simulink model "data_acq_passiveV2"  (R2016b)
settings: Solver=FixedStepDiscrete  StartTime=0.0  StopTime=300  FixedStep=.001  RelTol=1e-3  EnableMultiTasking=on
values from neighbouring files (symbols this model uses):
  offset = [0 0]    [Calibration_Run_Script.m]    (also in DAQ_Run_Script.m; bias.m = signal)
undefined symbols (not defined in the file or in its folder): bit, fdesignblkfcn, gcbh, Standard
libraries: slrtlib x11, xpclib x6, canmsglib x5, simulink x5, xpcnilib x3
(part 1 of 2)
settings Model: SimulationMode=external  Creator=localadmin  LastModifiedBy=1108gotthem
settings SolverCC: EnableConcurrentExecution=on  AutoInsertRateTranBlk=on
settings DataIOCC: SaveFormat=Structure  SignalLoggingSaveFormat=ModelDataLogs
settings OptimizationCC: BlockReduction=off  OptimizeBlockIOStorage=off  BufferReuse=off  GlobalBufferReuse=off  ExpressionFolding=off  ExpressionDepthLimit=2147483647  LocalBlockOutputs=off
settings DebuggingCC: UnderspecifiedInitializationDetection=Classic  MergeDetectMultiDrivingBlocksExec=none  SolverPrmCheckMsg=warning  FcnCallInpInsideContextMsg=warning  StateNameClashWarn=warning  SFUnexpectedBacktrackingDiag=warning  SFNoUnconditionalDefaultTransitionDiag=warning  SFExecutionAtInitializationDiag=none
settings HardwareCC: ProdBitPerPointer=32  ProdBitPerSizeT=32  ProdBitPerPtrDiffT=32  ProdLargestAtomicFloat=None  ProdWordSize=32  ProdLongLongMode=on  ProdHWDeviceType=Generic->32-bit x86 compatible
settings ModelReferenceCC: PropagateSignalLabelsOutOfModel=off
settings RTWCC: SystemTargetFile=slrt.tlc  TemplateMakefile=slrt_default_tmf  Description=Simulink Real-Time  RTWCompilerOptimization=on
settings SimulinkRealTimeCC: RL32LogBufSizeModifier=10200000  xPCIRQSourceBoard=Speedgoat_IO331
settings ConfigComp: CovMetricSettings=dw  CovHtmlReporting=on  CovSaveCumulativeToWorkspaceVar=on  CovSaveSingleToWorkspaceVar=on  CovExternalEMLEnable=off

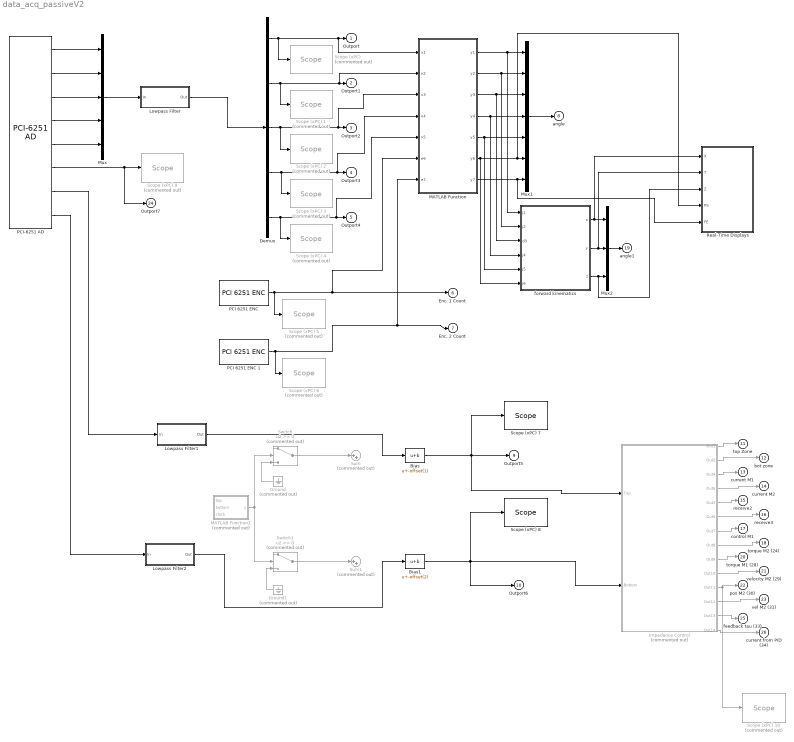
== system data_acq_passiveV2 ==
  Bias : Bias  Bias=-offset(1)
  Bias1 : Bias  Bias=-offset(2)
  Demux : Demux  Outputs=5
  Ground : Ground  Commented=on
  Ground1 : Ground  Commented=on
  Impedance Control : Subsystem  Commented=on
  Lowpass Filter : Subsystem  DialogController=fdesignblkfcn  InitFcn=fdesignblkfcn(gcbh, {'InitFcn'});  mask(Lowpass Filter){}
      mask help: Design a lowpass filter
      settings: CopyFcn=fdesignblkfcn(gcbh, {'CopyFcn'});
      mask Help: helpview(mapfilelocation('dsp'), 'dsplowpassfilter');
      mask Display: disp('Lowpass')
  Lowpass Filter1 : Subsystem  DialogController=fdesignblkfcn  InitFcn=fdesignblkfcn(gcbh, {'InitFcn'});  mask(Lowpass Filter){}
      mask help: Design a lowpass filter
      settings: CopyFcn=fdesignblkfcn(gcbh, {'CopyFcn'});
      mask Help: helpview(mapfilelocation('dsp'), 'dsplowpassfilter');
      mask Display: disp('Lowpass')
  Lowpass Filter2 : Subsystem  DialogController=fdesignblkfcn  InitFcn=fdesignblkfcn(gcbh, {'InitFcn'});  mask(Lowpass Filter){}
      mask help: Design a lowpass filter
      settings: CopyFcn=fdesignblkfcn(gcbh, {'CopyFcn'});
      mask Help: helpview(mapfilelocation('dsp'), 'dsplowpassfilter');
      mask Display: disp('Lowpass')
  MATLAB Function : MATLAB Function  TreatAsAtomicUnit=on
  MATLAB Function1 : MATLAB Function  Commented=on  TreatAsAtomicUnit=on
  Mux : Mux  Inputs=5
  Mux1 : Mux  Inputs=7
  Mux2 : Mux  Inputs=3
  "PCI 6251 ENC " : xpcnilib/Incremental Encoder/PCI 6251 ENC   channel=1  countMode=Quadrature Mode x4  initCount=0  reload=off  indexPhase=A low B low  filter=None  sampleTime=0.001  slot=-1
  PCI 6251 ENC 1 : xpcnilib/Incremental Encoder/PCI 6251 ENC   channel=0  countMode=Quadrature Mode x4  initCount=0  reload=off  indexPhase=A low B low  filter=None  sampleTime=0.001  slot=-1
  PCI-6251 AD : xpcnilib/A//D/M Series/PCI-6251 AD  channel=[1,2,3,4,5,6,7,8]  range=[10,10,10,10,10,10,10,10]  coupling=[1,1,1,1,1,1,2,2]  scantime=5e-6  sampletime=0.001  slot=-1
  "Real-Time Displays " : Subsystem
  "Scope (xPC) " : slrtlib/Displays and Logging/Scope   Commented=on  scopeno=6  scopetype=Target  autostart=on  viewmode=Graphical rolling  formatstr='%15.6f'  grid=on  ylimits=[7,10]  nosamples=15001  noprepostsamples=0  interleave=1  triggermode=FreeRun  triggersignal=1  trigsignalfromport=off  triggerlevel=0.0  triggerslope=Either  triggerscope=1  triggersample=0  filename=data.dat  mode=Lazy  writesize=512  autorestart=off  dynamicfilemode=off  maxwritefilesize=512*1024^2
  Scope (xPC) 1 : slrtlib/Displays and Logging/Scope   Commented=on  scopeno=1  scopetype=Target  autostart=on  viewmode=Graphical rolling  formatstr='%15.6f'  grid=on  ylimits=[5,9]  nosamples=15001  noprepostsamples=0  interleave=1  triggermode=FreeRun  triggersignal=1  trigsignalfromport=off  triggerlevel=0.0  triggerslope=Either  triggerscope=1  triggersample=0  filename=data.dat  mode=Lazy  writesize=512  autorestart=off  dynamicfilemode=off  maxwritefilesize=512*1024^2
  Scope (xPC) 10 : slrtlib/Displays and Logging/Scope   Commented=on  scopeno=5  scopetype=Target  autostart=on  viewmode=Graphical rolling  formatstr='%15.6f'  grid=on  ylimits=[-250,250]  nosamples=15001  noprepostsamples=0  interleave=1  triggermode=FreeRun  triggersignal=1  trigsignalfromport=off  triggerlevel=0.0  triggerslope=Either  triggerscope=1  triggersample=0  filename=data.dat  mode=Lazy  writesize=512  autorestart=off  dynamicfilemode=off  maxwritefilesize=512*1024^2
  Scope (xPC) 2 : slrtlib/Displays and Logging/Scope   Commented=on  scopeno=2  scopetype=Target  autostart=on  viewmode=Graphical rolling  formatstr='%15.6f'  grid=on  ylimits=[0,10]  nosamples=15001  noprepostsamples=0  interleave=1  triggermode=FreeRun  triggersignal=1  trigsignalfromport=off  triggerlevel=0.0  triggerslope=Either  triggerscope=1  triggersample=0  filename=data.dat  mode=Lazy  writesize=512  autorestart=off  dynamicfilemode=off  maxwritefilesize=512*1024^2
  Scope (xPC) 3 : slrtlib/Displays and Logging/Scope   Commented=on  scopeno=3  scopetype=Target  autostart=on  viewmode=Graphical rolling  formatstr='%15.6f'  grid=on  ylimits=[4.5,8.5]  nosamples=15001  noprepostsamples=0  interleave=1  triggermode=FreeRun  triggersignal=1  trigsignalfromport=off  triggerlevel=0.0  triggerslope=Either  triggerscope=1  triggersample=0  filename=data.dat  mode=Lazy  writesize=512  autorestart=off  dynamicfilemode=off  maxwritefilesize=512*1024^2
  Scope (xPC) 4 : slrtlib/Displays and Logging/Scope   Commented=on  scopeno=7  scopetype=Target  autostart=on  viewmode=Graphical rolling  formatstr='%15.6f'  grid=on  ylimits=[5,9]  nosamples=15001  noprepostsamples=0  interleave=1  triggermode=FreeRun  triggersignal=1  trigsignalfromport=off  triggerlevel=0.0  triggerslope=Either  triggerscope=1  triggersample=0  filename=data.dat  mode=Lazy  writesize=512  autorestart=off  dynamicfilemode=off  maxwritefilesize=512*1024^2
  Scope (xPC) 5 : slrtlib/Displays and Logging/Scope   Commented=on  scopeno=4  scopetype=Target  autostart=on  viewmode=Graphical rolling  formatstr='%15.6f'  grid=on  ylimits=[-15000,15000]  nosamples=15001  noprepostsamples=0  interleave=1  triggermode=FreeRun  triggersignal=1  trigsignalfromport=off  triggerlevel=0.0  triggerslope=Either  triggerscope=1  triggersample=0  filename=data.dat  mode=Lazy  writesize=512  autorestart=off  dynamicfilemode=off  maxwritefilesize=512*1024^2
  Scope (xPC) 6 : slrtlib/Displays and Logging/Scope   Commented=on  scopeno=5  scopetype=Target  autostart=on  viewmode=Graphical rolling  formatstr='%15.6f'  grid=on  ylimits=[-40000,40000]  nosamples=15001  noprepostsamples=0  interleave=1  triggermode=FreeRun  triggersignal=1  trigsignalfromport=off  triggerlevel=0.0  triggerslope=Either  triggerscope=1  triggersample=0  filename=data.dat  mode=Lazy  writesize=512  autorestart=off  dynamicfilemode=off  maxwritefilesize=512*1024^2
  Scope (xPC) 7 : slrtlib/Displays and Logging/Scope   scopeno=8  scopetype=Target  autostart=on  viewmode=Graphical rolling  formatstr='%15.6f'  grid=on  ylimits=[-1,1]  nosamples=20001  noprepostsamples=0  interleave=1  triggermode=FreeRun  triggersignal=1  trigsignalfromport=off  triggerlevel=0.0  triggerslope=Either  triggerscope=1  triggersample=0  filename=data.dat  mode=Lazy  writesize=512  autorestart=off  dynamicfilemode=off  maxwritefilesize=512*1024^2
  Scope (xPC) 8 : slrtlib/Displays and Logging/Scope   scopeno=9  scopetype=Target  autostart=on  viewmode=Graphical rolling  formatstr='%15.6f'  grid=on  ylimits=[-1,1]  nosamples=20001  noprepostsamples=0  interleave=1  triggermode=FreeRun  triggersignal=1  trigsignalfromport=off  triggerlevel=0.0  triggerslope=Either  triggerscope=1  triggersample=0  filename=data.dat  mode=Lazy  writesize=512  autorestart=off  dynamicfilemode=off  maxwritefilesize=512*1024^2
  Scope (xPC) 9 : slrtlib/Displays and Logging/Scope   Commented=on  scopeno=2  scopetype=Target  autostart=on  viewmode=Graphical rolling  formatstr='%15.6f'  grid=on  ylimits=[0,10]  nosamples=15001  noprepostsamples=0  interleave=1  triggermode=FreeRun  triggersignal=1  trigsignalfromport=off  triggerlevel=0.0  triggerslope=Either  triggerscope=1  triggersample=0  filename=data.dat  mode=Lazy  writesize=512  autorestart=off  dynamicfilemode=off  maxwritefilesize=512*1024^2
  Sum : Sum  Commented=on  Inputs=|++
  Sum1 : Sum  Commented=on  Inputs=|++
  Switch : Switch  Commented=on
  Switch1 : Switch  Commented=on
  forward kinematics : MATLAB Function  TreatAsAtomicUnit=on
  Outport : Outport  InitialOutput=0
  Outport1 : Outport  Port=2  InitialOutput=0
  Outport2 : Outport  Port=3  InitialOutput=0
  Outport3 : Outport  Port=4  InitialOutput=0
  Outport4 : Outport  Port=5  InitialOutput=0
  Enc. 1 Count : Outport  Port=6  InitialOutput=0
  Enc. 2 Count : Outport  Port=7  InitialOutput=0
  angle : Outport  Port=8  InitialOutput=0
  Outport5 : Outport  Port=9  InitialOutput=0
  Outport6 : Outport  Port=10  InitialOutput=0
  top Zone : Outport  Port=11  InitialOutput=0
  bot zone : Outport  Port=12  InitialOutput=0
  current M1 : Outport  Port=13  InitialOutput=0
  current M2 : Outport  Port=14  InitialOutput=0
  receive2 : Outport  Port=15  InitialOutput=0
  receive3 : Outport  Port=16  InitialOutput=0
  control M1 : Outport  Port=17  InitialOutput=0
  torque M2 (24) : Outport  Port=18  InitialOutput=0
  angle1 : Outport  Port=19  InitialOutput=0
  torque M1 (28) : Outport  Port=20  InitialOutput=0
  velocity M2 (29) : Outport  Port=21  InitialOutput=0
  pos M2 (30) : Outport  Port=22  InitialOutput=0
  vel M2 (31) : Outport  Port=23  InitialOutput=0
  Outport7 : Outport  Port=24  InitialOutput=0
  feedback tau (33) : Outport  Port=25  InitialOutput=0
  current from PID (34) : Outport  Port=26  InitialOutput=0
  wires:
  PCI-6251 AD/1 -> Mux/1
  PCI-6251 AD/2 -> Mux/2
  PCI-6251 AD/3 -> Mux/3
  PCI-6251 AD/4 -> Mux/4
  Demux/1 -> "Scope (xPC) "/1, MATLAB Function/1(v1), Outport/1
  Lowpass Filter/1(Out) -> Demux/1
  MATLAB Function/1(y1) -> forward kinematics/1(j1), Mux1/1
  MATLAB Function/2(y2) -> forward kinematics/2(j2), Mux1/2
  MATLAB Function/3(y3) -> forward kinematics/3(d3), Mux1/3
  MATLAB Function/4(y4) -> forward kinematics/4(j4), Mux1/4
  MATLAB Function/5(y5) -> forward kinematics/5(j5), Mux1/5
  Mux1/1 -> angle/1
  MATLAB Function/6(y6) -> forward kinematics/6(j6), "Real-Time Displays "/4(PS), Mux1/6
  MATLAB Function/7(y7) -> "Real-Time Displays "/5(FE), Mux1/7
  PCI-6251 AD/5 -> Mux/5
  Mux/1 -> Lowpass Filter/1(In)
  Demux/2 -> Scope (xPC) 1/1, MATLAB Function/2(v2), Outport1/1
  Demux/3 -> Scope (xPC) 2/1, MATLAB Function/3(v3), Outport2/1
  Demux/4 -> Scope (xPC) 3/1, MATLAB Function/4(v4), Outport3/1
  Demux/5 -> Scope (xPC) 4/1, Outport4/1, MATLAB Function/5(v5)
  PCI 6251 ENC 1/1 -> MATLAB Function/7(e7), Enc. 2 Count/1, Scope (xPC) 6/1
  "PCI 6251 ENC "/1 -> Scope (xPC) 5/1, MATLAB Function/6(e6), Enc. 1 Count/1
  Impedance Control/1(Out1) -> top Zone/1
  Impedance Control/2(Out2) -> bot zone/1
  Impedance Control/3(Out4) -> current M1/1
  Impedance Control/4(Out6) -> current M2/1
  Impedance Control/5(Out3) -> receive2/1
  Impedance Control/6(Out5) -> receive3/1
  Impedance Control/7(Out7) -> control M1/1
  Impedance Control/8(Out8) -> torque M2 (24)/1
  forward kinematics/1(x) -> "Real-Time Displays "/1(X), Mux2/1
  forward kinematics/2(y) -> "Real-Time Displays "/2(Y), Mux2/2
  forward kinematics/3(z) -> "Real-Time Displays "/3(Z), Mux2/3
  Mux2/1 -> angle1/1
  Impedance Control/9(Out9) -> torque M1 (28)/1
  Impedance Control/10(Out10) -> velocity M2 (29)/1
  Impedance Control/12(Out12) -> vel M2 (31)/1
  MATLAB Function1/1(y) -> Switch/2, Switch1/2
  Ground/1 -> Switch/3
  Switch/1 -> Sum/1
  Ground1/1 -> Switch1/3
  Switch1/1 -> Sum1/1
  Bias/1 -> Impedance Control/1(Top), Scope (xPC) 7/1, Outport5/1
  Bias1/1 -> Scope (xPC) 8/1, Outport6/1, Impedance Control/2(Bottom)
  PCI-6251 AD/6 -> Outport7/1, Scope (xPC) 9/1
  Impedance Control/11(Out11) -> Scope (xPC) 10/1, pos M2 (30)/1
  Impedance Control/13(Out13) -> feedback tau (33)/1
  Impedance Control/14(Out14) -> current from PID (34)/1
  PCI-6251 AD/7 -> Lowpass Filter1/1(In)
  Lowpass Filter1/1(Out) -> Bias/1
  PCI-6251 AD/8 -> Lowpass Filter2/1(In)
  Lowpass Filter2/1(Out) -> Bias1/1

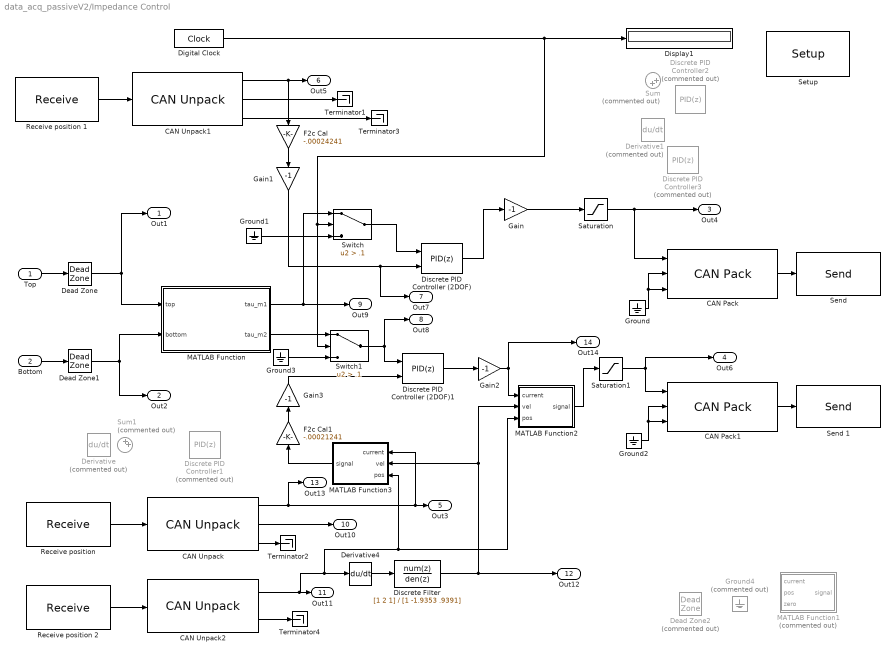
== system data_acq_passiveV2/Impedance Control ==
  Top : Inport
  Bottom : Inport  Port=2
  CAN Pack : canmsglib/CAN Pack  MsgList=(none)  MsgName=CAN Msg  MsgIDType=Standard (11-bit identifier)  MsgIdentifier=hex2dec('202')  MsgLength=8  SignalInfo=current$0$16$1$1$1$0$1$0$-Inf$Inf$#null$16$16$1$1$1$0$1$0$-Inf$Inf$#null2$32$32$1$1$1$0$1$0$-Inf$Inf$#  NSignals=3  StartBits=str2num('[int32(0);int32(16);int32(32)]')  SignalSizes=str2num('[int32(16);int32(16);int32(32)]')  ByteOrders=str2num('[int32(1);int32(1);int32(1)]')  DataTypes=str2num('[int32(1);int32(1);int32(1)]')  MultiplexTypes=str2num('[int32(1);int32(1);int32(1)]')  MultiplexValues=str2num('[double(0);double(0);double(0)]')  Factors=str2num('[double(1);double(1);double(1)]')  Offsets=str2num('[double(0);double(0);double(0)]')  Minimums=str2num('[double(-Inf);double(-Inf);double(-Inf)]')  Maximums=str2num('[double(Inf);double(Inf);double(Inf)]')  Remote=off
      settings: DataFormat=manually specified signals
  CAN Pack1 : canmsglib/CAN Pack  MsgList=(none)  MsgName=CAN Msg  MsgIDType=Standard (11-bit identifier)  MsgIdentifier=hex2dec('201')  MsgLength=8  SignalInfo=current$0$16$1$1$1$0$1$0$-Inf$Inf$#null$16$16$1$1$1$0$1$0$-Inf$Inf$#null2$32$32$1$1$1$0$1$0$-Inf$Inf$#  NSignals=3  StartBits=str2num('[int32(0);int32(16);int32(32)]')  SignalSizes=str2num('[int32(16);int32(16);int32(32)]')  ByteOrders=str2num('[int32(1);int32(1);int32(1)]')  DataTypes=str2num('[int32(1);int32(1);int32(1)]')  MultiplexTypes=str2num('[int32(1);int32(1);int32(1)]')  MultiplexValues=str2num('[double(0);double(0);double(0)]')  Factors=str2num('[double(1);double(1);double(1)]')  Offsets=str2num('[double(0);double(0);double(0)]')  Minimums=str2num('[double(-Inf);double(-Inf);double(-Inf)]')  Maximums=str2num('[double(Inf);double(Inf);double(Inf)]')  Remote=off
      settings: DataFormat=manually specified signals
  CAN Unpack : canmsglib/CAN Unpack  MsgList=(none)  MsgName=CAN Msg  MsgIDType=Standard (11-bit identifier)  MsgIdentifier=hex2dec('181')  MsgLength=8  SignalInfo=Current$0$16$1$1$1$0$1$0$-Inf$Inf$#vel$16$32$1$2$1$0$1$0$-Inf$Inf$#null2$48$16$1$1$1$0$1$0$-Inf$Inf$#  NSignals=3  IDPort=off  TimestampPort=off  ErrorPort=off  RemotePort=off  LengthPort=off  StatusPort=off  StartBits=str2num('[int32(0);int32(16);int32(48)]')  SignalSizes=str2num('[int32(16);int32(32);int32(16)]')  ByteOrders=str2num('[int32(1);int32(1);int32(1)]')  DataTypes=str2num('[int32(1);int32(2);int32(1)]')  MultiplexTypes=str2num('[int32(1);int32(1);int32(1)]')  MultiplexValues=str2num('[double(0);double(0);double(0)]')  Factors=str2num('[double(1);double(1);double(1)]')  Offsets=str2num('[double(0);double(0);double(0)]')  Minimums=str2num('[double(-Inf);double(-Inf);double(-Inf)]')  Maximums=str2num('[double(Inf);double(Inf);double(Inf)]')
  CAN Unpack1 : canmsglib/CAN Unpack  MsgList=(none)  MsgName=CAN Msg  MsgIDType=Standard (11-bit identifier)  MsgIdentifier=hex2dec('182')  MsgLength=8  SignalInfo=Current$0$16$1$1$1$0$1$0$-Inf$Inf$#null$16$32$1$2$1$0$1$0$-Inf$Inf$#null2$48$16$1$1$1$0$1$0$-Inf$Inf$#  NSignals=3  IDPort=off  TimestampPort=off  ErrorPort=off  RemotePort=off  LengthPort=off  StatusPort=off  StartBits=str2num('[int32(0);int32(16);int32(48)]')  SignalSizes=str2num('[int32(16);int32(32);int32(16)]')  ByteOrders=str2num('[int32(1);int32(1);int32(1)]')  DataTypes=str2num('[int32(1);int32(2);int32(1)]')  MultiplexTypes=str2num('[int32(1);int32(1);int32(1)]')  MultiplexValues=str2num('[double(0);double(0);double(0)]')  Factors=str2num('[double(1);double(1);double(1)]')  Offsets=str2num('[double(0);double(0);double(0)]')  Minimums=str2num('[double(-Inf);double(-Inf);double(-Inf)]')  Maximums=str2num('[double(Inf);double(Inf);double(Inf)]')
  CAN Unpack2 : canmsglib/CAN Unpack  MsgList=(none)  MsgName=CAN Msg  MsgIDType=Standard (11-bit identifier)  MsgIdentifier=hex2dec('281')  MsgLength=8  SignalInfo=pos$0$32$1$1$1$0$1$0$-Inf$Inf$#null$32$32$1$2$1$0$1$0$-Inf$Inf$#  NSignals=2  IDPort=off  TimestampPort=off  ErrorPort=off  RemotePort=off  LengthPort=off  StatusPort=off  StartBits=str2num('[int32(0);int32(32)]')  SignalSizes=str2num('[int32(32);int32(32)]')  ByteOrders=str2num('[int32(1);int32(1)]')  DataTypes=str2num('[int32(1);int32(2)]')  MultiplexTypes=str2num('[int32(1);int32(1)]')  MultiplexValues=str2num('[double(0);double(0)]')  Factors=str2num('[double(1);double(1)]')  Offsets=str2num('[double(0);double(0)]')  Minimums=str2num('[double(-Inf);double(-Inf)]')  Maximums=str2num('[double(Inf);double(Inf)]')
  Dead Zone : DeadZone  LowerValue=-.05  UpperValue=.05  SampleTime=.001  SaturateOnIntegerOverflow=on
  Dead Zone1 : DeadZone  LowerValue=-.05  UpperValue=.05  SampleTime=.001  SaturateOnIntegerOverflow=on
  Dead Zone2 : DeadZone  Commented=on  LowerValue=-4e4  UpperValue=4e4  SampleTime=.001  SaturateOnIntegerOverflow=on
  Derivative : Derivative  Commented=on
  Derivative1 : Derivative  Commented=on
  Derivative4 : Derivative
  Digital Clock : DigitalClock  SampleTime=.001
  Discrete Filter : DiscreteFilter  Numerator=[1 2 1]  Denominator=[1 -1.9353 .9391]  SampleTime=.001
  Discrete PID Controller (2DOF) : simulink/Continuous/PID Controller (2DOF)  Controller=PID  TimeDomain=Discrete-time  SampleTime=.001  IntegratorMethod=Forward Euler  FilterMethod=Forward Euler  Form=Parallel  P=-206.434175056882  I=-412868.350113764  D=0  N=100  b=1  c=1  InitialConditionSource=internal  InitialConditionForIntegrator=0  InitialConditionForFilter=0  ExternalReset=none  LimitOutput=off  UpperSaturationLimit=inf  LowerSaturationLimit=-inf  LinearizeAsGain=off  AntiWindupMode=none  Kb=1  TrackingMode=off  Kt=1  PParamMin=[]  PParamMax=[]  IParamMin=[]  IParamMax=[]  DParamMin=[]  DParamMax=[]  NParamMin=[]  NParamMax=[]  bParamMin=[]  bParamMax=[]  cParamMin=[]  cParamMax=[]  KbParamMin=[]  KbParamMax=[]  KtParamMin=[]  KtParamMax=[]  POutMin=[]  POutMax=[]  IOutMin=[]  IOutMax=[]  DOutMin=[]  DOutMax=[]  NOutMin=[]  NOutMax=[]  bOutMin=[]  bOutMax=[]  cOutMin=[]  cOutMax=[]  KbOutMin=[]  KbOutMax=[]  KtOutMin=[]  KtOutMax=[]  IntegratorOutMin=[]  IntegratorOutMax=[]  FilterOutMin=[]  FilterOutMax=[]  SumOutMin=[]  SumOutMax=[]  Sum1OutMin=[]  Sum1OutMax=[]  Sum2OutMin=[]  Sum2OutMax=[]  Sum3OutMin=[]  Sum3OutMax=[]  SumI1OutMin=[]  SumI1OutMax=[]  SumI2OutMin=[]  SumI2OutMax=[]  SumI3OutMin=[]  SumI3OutMax=[]  SumDOutMin=[]  SumDOutMax=[]  SaturationOutMin=[]  SaturationOutMax=[]  IntegratorContinuousStateAttributes=''  IntegratorStateMustResolveToSignalObject=off  IntegratorRTWStateStorageClass=Auto  FilterContinuousStateAttributes=''  FilterStateMustResolveToSignalObject=off  FilterRTWStateStorageClass=Auto
  Discrete PID Controller (2DOF)1 : simulink/Continuous/PID Controller (2DOF)  Controller=PID  TimeDomain=Discrete-time  SampleTime=.001  IntegratorMethod=Forward Euler  FilterMethod=Forward Euler  Form=Parallel  P=-235.590171722324  I=-471180.343444648  D=0  N=100  b=1  c=1  InitialConditionSource=internal  InitialConditionForIntegrator=0  InitialConditionForFilter=0  ExternalReset=none  LimitOutput=off  UpperSaturationLimit=inf  LowerSaturationLimit=-inf  LinearizeAsGain=off  AntiWindupMode=none  Kb=1  TrackingMode=off  Kt=1  PParamMin=[]  PParamMax=[]  IParamMin=[]  IParamMax=[]  DParamMin=[]  DParamMax=[]  NParamMin=[]  NParamMax=[]  bParamMin=[]  bParamMax=[]  cParamMin=[]  cParamMax=[]  KbParamMin=[]  KbParamMax=[]  KtParamMin=[]  KtParamMax=[]  POutMin=[]  POutMax=[]  IOutMin=[]  IOutMax=[]  DOutMin=[]  DOutMax=[]  NOutMin=[]  NOutMax=[]  bOutMin=[]  bOutMax=[]  cOutMin=[]  cOutMax=[]  KbOutMin=[]  KbOutMax=[]  KtOutMin=[]  KtOutMax=[]  IntegratorOutMin=[]  IntegratorOutMax=[]  FilterOutMin=[]  FilterOutMax=[]  SumOutMin=[]  SumOutMax=[]  Sum1OutMin=[]  Sum1OutMax=[]  Sum2OutMin=[]  Sum2OutMax=[]  Sum3OutMin=[]  Sum3OutMax=[]  SumI1OutMin=[]  SumI1OutMax=[]  SumI2OutMin=[]  SumI2OutMax=[]  SumI3OutMin=[]  SumI3OutMax=[]  SumDOutMin=[]  SumDOutMax=[]  SaturationOutMin=[]  SaturationOutMax=[]  IntegratorContinuousStateAttributes=''  IntegratorStateMustResolveToSignalObject=off  IntegratorRTWStateStorageClass=Auto  FilterContinuousStateAttributes=''  FilterStateMustResolveToSignalObject=off  FilterRTWStateStorageClass=Auto
  Discrete PID Controller1 : simulink/Continuous/PID Controller  Commented=on  Controller=PID  TimeDomain=Discrete-time  SampleTime=.001  IntegratorMethod=Forward Euler  FilterMethod=Forward Euler  Form=Parallel  P=-1.8  I=-4000  D=0  N=100  InitialConditionSource=internal  InitialConditionForIntegrator=0  InitialConditionForFilter=0  ExternalReset=none  LimitOutput=off  UpperSaturationLimit=inf  LowerSaturationLimit=-inf  LinearizeAsGain=off  AntiWindupMode=none  Kb=1  TrackingMode=off  Kt=1  PParamMin=[]  PParamMax=[]  IParamMin=[]  IParamMax=[]  DParamMin=[]  DParamMax=[]  NParamMin=[]  NParamMax=[]  KbParamMin=[]  KbParamMax=[]  KtParamMin=[]  KtParamMax=[]  POutMin=[]  POutMax=[]  IOutMin=[]  IOutMax=[]  DOutMin=[]  DOutMax=[]  NOutMin=[]  NOutMax=[]  KbOutMin=[]  KbOutMax=[]  KtOutMin=[]  KtOutMax=[]  IntegratorOutMin=[]  IntegratorOutMax=[]  FilterOutMin=[]  FilterOutMax=[]  SumOutMin=[]  SumOutMax=[]  SumI1OutMin=[]  SumI1OutMax=[]  SumI2OutMin=[]  SumI2OutMax=[]  SumI3OutMin=[]  SumI3OutMax=[]  SumDOutMin=[]  SumDOutMax=[]  SaturationOutMin=[]  SaturationOutMax=[]  IntegratorContinuousStateAttributes=''  IntegratorStateMustResolveToSignalObject=off  IntegratorRTWStateStorageClass=Auto  FilterContinuousStateAttributes=''  FilterStateMustResolveToSignalObject=off  FilterRTWStateStorageClass=Auto
  Discrete PID Controller2 : simulink/Continuous/PID Controller  Commented=on  Controller=PID  TimeDomain=Discrete-time  SampleTime=.001  IntegratorMethod=Forward Euler  FilterMethod=Forward Euler  Form=Parallel  P=10  I=500  D=2  N=1  InitialConditionSource=internal  InitialConditionForIntegrator=0  InitialConditionForFilter=0  ExternalReset=none  LimitOutput=off  UpperSaturationLimit=inf  LowerSaturationLimit=-inf  LinearizeAsGain=off  AntiWindupMode=none  Kb=1  TrackingMode=off  Kt=1  PParamMin=[]  PParamMax=[]  IParamMin=[]  IParamMax=[]  DParamMin=[]  DParamMax=[]  NParamMin=[]  NParamMax=[]  KbParamMin=[]  KbParamMax=[]  KtParamMin=[]  KtParamMax=[]  POutMin=[]  POutMax=[]  IOutMin=[]  IOutMax=[]  DOutMin=[]  DOutMax=[]  NOutMin=[]  NOutMax=[]  KbOutMin=[]  KbOutMax=[]  KtOutMin=[]  KtOutMax=[]  IntegratorOutMin=[]  IntegratorOutMax=[]  FilterOutMin=[]  FilterOutMax=[]  SumOutMin=[]  SumOutMax=[]  SumI1OutMin=[]  SumI1OutMax=[]  SumI2OutMin=[]  SumI2OutMax=[]  SumI3OutMin=[]  SumI3OutMax=[]  SumDOutMin=[]  SumDOutMax=[]  SaturationOutMin=[]  SaturationOutMax=[]  IntegratorContinuousStateAttributes=''  IntegratorStateMustResolveToSignalObject=off  IntegratorRTWStateStorageClass=Auto  FilterContinuousStateAttributes=''  FilterStateMustResolveToSignalObject=off  FilterRTWStateStorageClass=Auto
  Discrete PID Controller3 : simulink/Continuous/PID Controller  Commented=on  Controller=PID  TimeDomain=Discrete-time  SampleTime=.001  IntegratorMethod=Forward Euler  FilterMethod=Forward Euler  Form=Parallel  P=-1.8  I=-4000  D=0  N=100  InitialConditionSource=internal  InitialConditionForIntegrator=0  InitialConditionForFilter=0  ExternalReset=none  LimitOutput=off  UpperSaturationLimit=inf  LowerSaturationLimit=-inf  LinearizeAsGain=off  AntiWindupMode=none  Kb=1  TrackingMode=off  Kt=1  PParamMin=[]  PParamMax=[]  IParamMin=[]  IParamMax=[]  DParamMin=[]  DParamMax=[]  NParamMin=[]  NParamMax=[]  KbParamMin=[]  KbParamMax=[]  KtParamMin=[]  KtParamMax=[]  POutMin=[]  POutMax=[]  IOutMin=[]  IOutMax=[]  DOutMin=[]  DOutMax=[]  NOutMin=[]  NOutMax=[]  KbOutMin=[]  KbOutMax=[]  KtOutMin=[]  KtOutMax=[]  IntegratorOutMin=[]  IntegratorOutMax=[]  FilterOutMin=[]  FilterOutMax=[]  SumOutMin=[]  SumOutMax=[]  SumI1OutMin=[]  SumI1OutMax=[]  SumI2OutMin=[]  SumI2OutMax=[]  SumI3OutMin=[]  SumI3OutMax=[]  SumDOutMin=[]  SumDOutMax=[]  SaturationOutMin=[]  SaturationOutMax=[]  IntegratorContinuousStateAttributes=''  IntegratorStateMustResolveToSignalObject=off  IntegratorRTWStateStorageClass=Auto  FilterContinuousStateAttributes=''  FilterStateMustResolveToSignalObject=off  FilterRTWStateStorageClass=Auto
  Display1 : Display
      settings: Format=hex (Stored Integer)
  F2c Cal : Gain  Gain=-.00024241  SampleTime=.001
  F2c Cal1 : Gain  Gain=-.00021241  SampleTime=.001
  Gain{,1..3} (4 alike) : Gain  Gain=-1
  Ground{,1..3} (4 alike) : Ground
  Ground4 : Ground  Commented=on
  MATLAB Function : MATLAB Function  TreatAsAtomicUnit=on
  MATLAB Function1 : MATLAB Function  Commented=on  TreatAsAtomicUnit=on
  MATLAB Function2 : MATLAB Function  TreatAsAtomicUnit=on
  MATLAB Function3 : MATLAB Function  TreatAsAtomicUnit=on
  "Receive position " : xpclib/CAN/Softing/CAN-AC2-PCI SJA 1000/Receive   board=1  canPort=CAN 1  range=Standard (11-bit)  ids=hex2dec('181')  lengths=8  output=CAN_MESSAGE data type  inten=off  ts=0.001  ididx=[0]
  Receive position 1 : xpclib/CAN/Softing/CAN-AC2-PCI SJA 1000/Receive   board=1  canPort=CAN 1  range=Standard (11-bit)  ids=hex2dec('182')  lengths=8  output=CAN_MESSAGE data type  inten=off  ts=0.001  ididx=[1]
  Receive position 2 : xpclib/CAN/Softing/CAN-AC2-PCI SJA 1000/Receive   board=1  canPort=CAN 1  range=Standard (11-bit)  ids=hex2dec('281')  lengths=8  output=CAN_MESSAGE data type  inten=off  ts=0.001  ididx=[2]
  Saturation : Saturate  UpperLimit=1700  LowerLimit=-1700  LinearizeAsGain=off  SampleTime=.001
  Saturation1 : Saturate  UpperLimit=1700  LowerLimit=-1700  LinearizeAsGain=off
  "Send " : xpclib/CAN/Softing/CAN-AC2-PCI SJA 1000/Send   board=1  canPort=CAN 1  range=Standard (11-bit)  ids=hex2dec('202')  sizes=[8]  output=off  ts=0.001  ididx=[2]
  Send 1 : xpclib/CAN/Softing/CAN-AC2-PCI SJA 1000/Send   board=1  canPort=CAN 1  range=Standard (11-bit)  ids=hex2dec('201')  sizes=[8]  output=off  ts=0.001  ididx=[1]
  "Setup " : xpclib/CAN/Softing/CAN-AC2-PCI SJA 1000/Setup   board=1  can1bus=Highspeed (ISO 11898)  can1Baudrate=1 MBaud  can1UserBR=[1,1,4,3]  can2bus=Highspeed (ISO 11898)  can2Baudrate=1 MBaud  can2UserBR=[1,1,4,3]  init=pdo_start  term=pdo_stop  bus_off_out=off  bus_off_rec=Off  ioBaseAddress=-1
  Sum : Sum  Commented=on  Inputs=|++
  Sum1 : Sum  Commented=on  Inputs=|++
  Switch : Switch  Criteria=u2 > Threshold  Threshold=.1  SampleTime=.001
  Switch1 : Switch  Criteria=u2 > Threshold  Threshold=.1
  Terminator{1..4} (4 alike) : Terminator
  Out1 : Outport
  Out2 : Outport  Port=2
  Out4 : Outport  Port=3
  Out6 : Outport  Port=4
  Out3 : Outport  Port=5
  Out5 : Outport  Port=6
  Out7 : Outport  Port=7
  Out8 : Outport  Port=8
  Out9 : Outport  Port=9
  Out10 : Outport  Port=10
  Out11 : Outport  Port=11
  Out12 : Outport  Port=12
  Out13 : Outport  Port=13
  Out14 : Outport  Port=14
  wires:
  Ground/1 -> CAN Pack/2, CAN Pack/3
  CAN Pack/1 -> "Send "/1
  "Receive position "/1 -> CAN Unpack/1
  CAN Unpack/2 -> Out10/1
  CAN Unpack/1 -> Out13/1, MATLAB Function3/1(current), Out3/1
  Digital Clock/1 -> Display1/1, Switch1/2, Switch/2
  Dead Zone/1 -> MATLAB Function/1(top), Out1/1
  Dead Zone1/1 -> Out2/1, MATLAB Function/2(bottom)
  Ground2/1 -> CAN Pack1/2, CAN Pack1/3
  CAN Pack1/1 -> Send 1/1
  MATLAB Function/2(tau_m2) -> Switch1/1
  CAN Unpack1/1 -> F2c Cal/1, Out5/1
  CAN Unpack1/2 -> Terminator1/1
  Receive position 1/1 -> CAN Unpack1/1
  CAN Unpack1/3 -> Terminator3/1
  CAN Unpack/3 -> Terminator2/1
  Top/1 -> Dead Zone/1
  Bottom/1 -> Dead Zone1/1
  MATLAB Function/1(tau_m1) -> Switch/1, Out9/1
  Discrete PID Controller (2DOF)/1 -> Gain/1
  Discrete PID Controller (2DOF)1/1 -> Gain2/1
  F2c Cal/1 -> Gain1/1
  F2c Cal1/1 -> Gain3/1
  Gain/1 -> Saturation/1
  Gain1/1 -> Out7/1, Discrete PID Controller (2DOF)/2
  Gain3/1 -> Discrete PID Controller (2DOF)1/2
  Receive position 2/1 -> CAN Unpack2/1
  CAN Unpack2/2 -> Terminator4/1
  Derivative4/1 -> Discrete Filter/1
  Discrete Filter/1 -> MATLAB Function3/2(vel), MATLAB Function2/2(vel), Out12/1
  Saturation1/1 -> Out6/1, CAN Pack1/1
  Saturation/1 -> Out4/1, CAN Pack/1
  Ground1/1 -> Switch/3
  Switch/1 -> Discrete PID Controller (2DOF)/1
  Switch1/1 -> Out8/1, Discrete PID Controller (2DOF)1/1
  Ground3/1 -> Switch1/3
  CAN Unpack2/1 -> MATLAB Function3/3(pos), MATLAB Function2/3(pos), Derivative4/1, Out11/1
  MATLAB Function3/1(signal) -> F2c Cal1/1
  MATLAB Function2/1(signal) -> Saturation1/1
  Gain2/1 -> MATLAB Function2/1(current), Out14/1

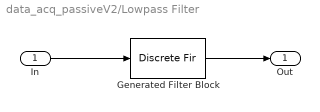
== system data_acq_passiveV2/Lowpass Filter ==
  In : Inport
  Generated Filter Block : DiscreteFir  Tag=BlockMethodSubSystem  Coefficients=[-0.00052324228244352597 -5.6057008840111622e-05 -5.9029960060090123e-05 -6.2089092415703651e-05 -6.5235172106602808e-05 -6.8468792239146433e-05 -7.1791170876184978e-05 -7.5199394031231657e-05 -7.8693485466635764e-05 -8.2278777605507031e-05 -8.595347305185517e-05 -8.9721309412065051e-05 -9.3578658035005043e-05 -9.7527959693077641e-05 -0.00010156823183841502 -0.00010570306844346472 -0.0001099328592674625 -0.00011425592773425428 -0.00011867203248127299 -0.0001231799968737532 -0.00012778728307383345 -0.00013249067611977418 -0.00013729314500949554 -0.00014218232070427767 -0.00014716926331734948 -0.00015225602378782298 -0.00015743218992457042 -0.00016269728987213943 -0.00016806238974750827 -0.00017352033232048865 -0.0001790541571821037 -0.00018469470695856038 -0.00019040984292100611 -0.00019621615780973255 -0.00020210453549572777 -0.00020807769136475324 -0.00021413162898923835 -0.00022026741549891577 -0.00022648545623399775 -0.00023278305632693007 -0.00023916116470940019 -0.00024561752902621861 -0.00025215563189431487 -0.00025877239732060919 -0.00026546870783869639 -0.00027224140486980879 -0.00027909126326666029 -0.00028601702953346975 -0.00029301423418495693 -0.0003000833632016655 -0.00030721562663037119 -0.00031442057334346384 -0.00032166470362155413 -0.0003289859106662829 -0.00033634358815721359 -0.00034374313095350431 -0.00035119427093453651 -0.00035868375459999696 -0.0003662039702031097 -0.00037376552352817309 -0.0003813735840803234 -0.00038901495643876518 -0.00039669544877577199 -0.00040441363753715757 -0.00041217530568567532 -0.00041997236920575794 -0.00042779681226945903 -0.00043563648316667354 -0.00044348025734073965 -0.00045131682050124572 -0.00045913146718169523 -0.00046691658695320793 -0.00047466786789203153 -0.00048240036364918733 -0.00049013557695491749 -0.00049790927995173621 -0.00050574222671454687 -0.00051362605492419008 -0.00052149568150616993 -0.00052920115935022743 -0.00053654954320442034 -0.00054357771054403859 -0.00055214790105943346 -0.00055916535223403136 -0.00056666427607138812 -0.00057404465564137052 -0.00058135307459826859 -0.00058858746107408311 -0.00059574654644921473 -0.00060282347017059977 -0.00060981028743565169 -0.00061670493558216505 -0.00062349928924097396 -0.000630192055063267 -0.00063677471765257723 -0.00064324342516180089 -0.00064958972288984044 -0.00065581029697547931 -0.0006619013208642088 -0.00066785686227762093 -0.00067367026968544099 -0.00067932944837409447 -0.00068483347458354069 -0.00069017350542580796 -0.00069535230042428028 -0.00070034879032750846 -0.00070516462522351693 -0.00070979980509052972 -0.00071424020173444002 -0.00071847608015420902 -0.00072251270665083943 -0.00072634337800568096 -0.00072994321245200037 -0.00073333574344273337 -0.00073649156348525686 -0.00073941703893840895 -0.00074210053887124113 -0.00074453916177031048 -0.00074672281031526401 -0.00074864519360783878 -0.00075030132489939145 -0.00075168278519708134 -0.00075278399298329122 -0.00075359502155582811 -0.00075411336084044384 -0.00075433142515719212 -0.00075424619678480674 -0.00075384983500808959 -0.00075313851527801946 -0.0007521083156189119 -0.0007507511200035438 -0.00074906499149087695 -0.00074703433019716707 -0.00074467569886822607 -0.00074193430250794738 -0.00073886247530116969 -0.00073541239059260954 -0.00073157897963701992 -0.0007273769919590344 -0.00072279421000670443 -0.00071781259232127099 -0.00071243669254971711 -0.00070667704483942564 -0.00070052009746154594 -0.00069396076402879247 -0.00068698617116579529 -0.00067959495504656586 -0.00067177723621101009 -0.00066352416222824231 -0.0006548251523169538 -0.00064567650220373897 -0.00063608395400448962 -0.00062605373231083893 -0.00061559312159697338 -0.00060469234669886644 -0.00059333532482305806 -0.00058149012821433687 -0.00056914033755682623 -0.00055628848147566494 -0.00054297275957292416 -0.00052924873470221775 -0.00051510617355876131 -0.0005003889172763155 -0.00048493969539900724 -0.00046944146128394216 -0.00045313869696779349 -0.0004364405176052949 ...(+12253 chars)]
  Out : Outport
  wires:
  In/1 -> Generated Filter Block/1
  Generated Filter Block/1 -> Out/1

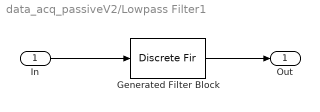
== system data_acq_passiveV2/Lowpass Filter1 ==
  In : Inport
  Generated Filter Block : DiscreteFir  Tag=BlockMethodSubSystem  Coefficients=[0.0035257793515495774 0.0038119531647798038 0.0041036148788394806 0.0044003780267683791 0.0047018389448218933 0.0050075775498282637 0.0053171581667394901 0.0056301304044040169 0.0059460300774376931 0.0062643801719234971 0.0065846918525311708 0.0069064655085147161 0.0072291918359202803 0.0075523529532183957 0.0078754235474644951 0.0081978720479896055 0.008519161824529782 0.008838752406618456 0.0091561007209909322 0.0094706623436844779 0.0097818927634617959 0.010089248653139572 0.010392189145368247 0.010690177109383412 0.010982680425234054 0.011269173251988259 0.011549137286422439 0.011822063008716528 0.012087450911703952 0.012344812710262444 0.01259367252747858 0.012833568054276996 0.013064051679271809 0.013284691585675896 0.013495072812189788 0.013694798274888394 0.013883489747229208 0.014060788795419015 0.014226357666499202 0.014379880126639598 0.014521062247269227 0.014649633136817507 0.014765345615991476 0.014867976834673335 0.014957328828686459 0.015033229014848307 0.015095530622902396 0.015144113063101152 0.015178882228393269 0.015199770730355538 0.015206738068197194 0.015199770730355538 0.015178882228393269 0.015144113063101152 0.015095530622902396 0.015033229014848307 0.014957328828686459 0.014867976834673335 0.014765345615991476 0.014649633136817507 0.014521062247269227 0.014379880126639598 0.014226357666499202 0.014060788795419015 0.013883489747229208 0.013694798274888394 0.013495072812189788 0.013284691585675896 0.013064051679271809 0.012833568054276996 0.01259367252747858 0.012344812710262444 0.012087450911703952 0.011822063008716528 0.011549137286422439 0.011269173251988259 0.010982680425234054 0.010690177109383412 0.010392189145368247 0.010089248653139572 0.0097818927634617959 0.0094706623436844779 0.0091561007209909322 0.008838752406618456 0.008519161824529782 0.0081978720479896055 0.0078754235474644951 0.0075523529532183957 0.0072291918359202803 0.0069064655085147161 0.0065846918525311708 0.0062643801719234971 0.0059460300774376931 0.0056301304044040169 0.0053171581667394901 0.0050075775498282637 0.0047018389448218933 0.0044003780267683791 0.0041036148788394806 0.0038119531647798038 0.0035257793515495774]  InputProcessing=Columns as channels (frame based)
  Out : Outport
  wires:
  In/1 -> Generated Filter Block/1
  Generated Filter Block/1 -> Out/1
